simulink model "three_level_sv"  (R2025a)
settings: Solver=ode1be  StartTime=0.0  StopTime=simlength  FixedStep=ts_sim  MaxStep=ts_sim
undefined symbols (not defined in the file): fPWM_INV, number_of_cells, Q, q1Kalman, q2Kalman, q3Kalman, rKalman, tc, ts_afe, ts_zvs, tsample, Vbattery_nom
libraries: fl_lib x118, nesl_utility x60, ee_lib x3, spsPWMGenerator3LevelLib x3, lithium_ion_cell_lib x2, simulink x2
(part 1 of 4)
settings Model: SimulationMode=accelerator  Creator=LTNBDA  LastModifiedBy=dbagn
settings SolverCC: ZeroCrossControl=EnableAll  ZeroCrossAlgorithm=Adaptive  AlgebraicLoopSolver=TrustRegion  SolverResetMethod=Robust  AutoInsertRateTranBlk=on
settings DataIOCC: LimitDataPoints=on  MaxDataPoints=1  SaveFormat=Array  SignalLoggingSaveFormat=ModelDataLogs  SaveOutput=off  SignalLogging=off  DSMLogging=off  SaveTime=off  ReturnWorkspaceOutputs=off
settings OptimizationCC: ExpressionDepthLimit=2147483647.0  InitFltsAndDblsToZero=on  EfficientMapNaN2IntZero=off  LifeSpan=inf
settings DebuggingCC: SaveWithParameterizedLinksMsg=none  UnderspecifiedInitializationDetection=Classic  MergeDetectMultiDrivingBlocksExec=none  SignalResolutionControl=TryResolveAllWithWarning  SolverPrmCheckMsg=warning  MultiTaskDSMMsg=warning  MultiTaskCondExecSysMsg=none  MultiTaskRateTransMsg=warning  FcnCallInpInsideContextMsg=warning  StateNameClashWarn=warning  SFUnexpectedBacktrackingDiag=warning  SFNoUnconditionalDefaultTransitionDiag=warning  ArithmeticOperatorsInVariantConditions=warning
settings HardwareCC: ProdBitPerLong=64.0  ProdLargestAtomicFloat=None  ProdIntDivRoundTo=Undefined  ProdEndianess=Unspecified  ProdHWDeviceType=Generic->64-bit Embedded Processor (LP64)  TargetBitPerPointer=64.0  TargetBitPerSizeT=64.0  TargetBitPerPtrDiffT=64.0  TargetLongLongMode=on  TargetIntDivRoundTo=Zero  TargetEndianess=LittleEndian  TargetWordSize=64.0  TargetHWDeviceType=MATLAB Host  ProdEqTarget=off
settings ModelReferenceCC: EnableRefExpFcnMdlSchedulingChecks=on  PropagateSignalLabelsOutOfModel=off
settings SFSimCC: SimUseLocalCustomCode=off  CustomCodeUndefinedFunction=UseInterfaceOnly
settings RTWCC: RTWUseLocalCustomCode=off  GPUComputeCapability=3.5
settings CodeAppCC: MaxIdLength=128.0  StateflowObjectComments=on
settings GRTTargetCC: TargetLangStandard=C89/C90 (ANSI)  CombineOutputUpdateFcns=off  GRTInterface=on
settings ConfigComp: CovMetricSettings=dw  CovSaveCumulativeToWorkspaceVar=on  CovSaveSingleToWorkspaceVar=on  CovExternalEMLEnable=off
settings SimscapeCC: SimscapeNormalizeSystem=off

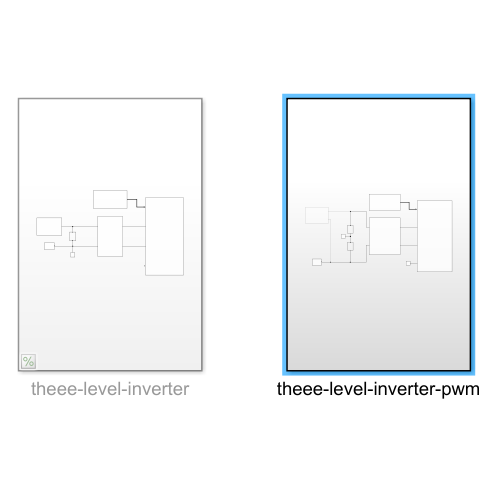
[thumbnail: Simulink's stored preview of the top-level diagram]
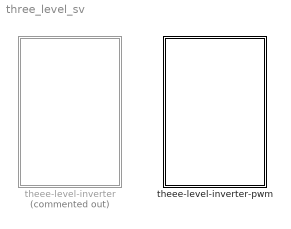
== system three_level_sv ==
  theee-level-inverter : Subsystem  Commented=on
  theee-level-inverter-pwm : Subsystem

== system three_level_sv/theee-level-inverter ==
  Electrical Reference2 : fl_lib/Electrical/Electrical Elements/Electrical Reference
  Solver Configuration : nesl_utility/Solver Configuration  PhysicalDomain=network_engine_domain  SubClassName=solver  LeftPortType=input  RightPortType=generic  Tones=[]  Harmonics=[]  SimulateNoise=off  Profile=off  UseLocalSampling=off  EnableSwitchedLinearOptims=on  FrequencyDomain=off  UseCCode=off  RelTol=0.001  AbsTol=0.001  MinStep=1e-09  ToWorkspace=off  RevertToSquareIcSolve=off  NumHomotopyIterations=100  PhasorMode=off  PhasorModeNumHarmonics=1  ConsistencySolver=NEWTON_FTOL  IndexReductionMethod=DerivativeReplacement  DoDC=on  ResidualTolerance=1e-09  ConsistencyTolSource=GLOBAL  ConsistencyAbsTol=0.001  ConsistencyRelTol=0.001  ConsistencyTolFactor=0.001  UseLocalSolver=on  LocalSolverChoice=NE_BACKWARD_EULER_ADVANCER  ResolveIndetEquations=on  FunctionEvalNumThread=1  LocalSolverSampleTime=ts_sim  DoFixedCost=on  MaxNonlinIter=3  MaxModeIter=2  ComputeImpulses=off  ImpulseIterations=2  LinearAlgebra=auto  LinearAlgebraNumThread=0  EquationFormulation=NE_TIME_EF  DelaysMemoryBudget=1024  AutomaticFiltering=on  FilteringTimeConstant=0.001  PartitionStorageMethod=AS_NEEDED  PartitionMemoryBudget=1024  PartitionMethod=ROBUST  MultibodyUseLocalSolver=off  MultibodyLocalSolverChoice=ODE1  MultibodyLocalSolverSampleTime=0.001
  Voltage Source : ee_lib/Sources/Voltage Source  dc_voltage=Vbattery_nom V  ac_voltage=0 V  ac_shift=0 rad  ac_frequency=60 Hz  noise_mode=ee.enum.sources.noise.Disabled  PSD=0 V^2/Hz  sample_time=1e-3 s  repeatability=ee.enum.sources.repeatability.NotRepeatable  user_seed=0  auto_seed=3499211588  i_specify=off  i_priority=None  i=0 A  i_nominal_specify=off  i_nominal_value=1  i_nominal_unit=A  v_specify=off  v_priority=None  v=0 V  v_nominal_specify=off  v_nominal_value=1  v_nominal_unit=V
  battery_system : Subsystem
  pwm_commands : Subsystem
  single_phase_ui_measure1 : Subsystem
  three-level-inverter : Subsystem
  wires:
  pwm_commands/1(gate_commands) -> three-level-inverter/1(gate_commands)
  connections:
  three-level-inverter/LConn2 -- single_phase_ui_measure1/RConn2
  battery_system/RConn1 -- Voltage Source/LConn1 -- single_phase_ui_measure1/LConn1
  single_phase_ui_measure1/RConn1 -- three-level-inverter/LConn1
  single_phase_ui_measure1/LConn2 -- Electrical Reference2/LConn1 -- Voltage Source/RConn1 -- Solver Configuration/RConn1

== system three_level_sv/theee-level-inverter-pwm ==
  Electrical Reference1 : fl_lib/Electrical/Electrical Elements/Electrical Reference
  Electrical Reference2 : fl_lib/Electrical/Electrical Elements/Electrical Reference
  Solver Configuration : nesl_utility/Solver Configuration  PhysicalDomain=network_engine_domain  SubClassName=solver  LeftPortType=input  RightPortType=generic  Tones=[]  Harmonics=[]  SimulateNoise=off  Profile=off  UseLocalSampling=off  EnableSwitchedLinearOptims=on  FrequencyDomain=off  UseCCode=off  RelTol=0.001  AbsTol=0.001  MinStep=1e-09  ToWorkspace=off  RevertToSquareIcSolve=off  NumHomotopyIterations=100  PhasorMode=off  PhasorModeNumHarmonics=1  ConsistencySolver=NEWTON_FTOL  IndexReductionMethod=DerivativeReplacement  DoDC=on  ResidualTolerance=1e-09  ConsistencyTolSource=GLOBAL  ConsistencyAbsTol=0.001  ConsistencyRelTol=0.001  ConsistencyTolFactor=0.001  UseLocalSolver=on  LocalSolverChoice=NE_BACKWARD_EULER_ADVANCER  ResolveIndetEquations=on  FunctionEvalNumThread=1  LocalSolverSampleTime=ts_sim  DoFixedCost=on  MaxNonlinIter=3  MaxModeIter=2  ComputeImpulses=off  ImpulseIterations=2  LinearAlgebra=auto  LinearAlgebraNumThread=0  EquationFormulation=NE_TIME_EF  DelaysMemoryBudget=1024  AutomaticFiltering=on  FilteringTimeConstant=0.001  PartitionStorageMethod=AS_NEEDED  PartitionMemoryBudget=1024  PartitionMethod=ROBUST  MultibodyUseLocalSolver=off  MultibodyLocalSolverChoice=ODE1  MultibodyLocalSolverSampleTime=0.001
  Voltage Source : ee_lib/Sources/Voltage Source  dc_voltage=Vbattery_nom/2 V  ac_voltage=0 V  ac_shift=0 rad  ac_frequency=60 Hz  noise_mode=ee.enum.sources.noise.Disabled  PSD=0 V^2/Hz  sample_time=1e-3 s  repeatability=ee.enum.sources.repeatability.NotRepeatable  user_seed=0  auto_seed=3499211588  i_specify=off  i_priority=None  i=0 A  i_nominal_specify=off  i_nominal_value=1  i_nominal_unit=A  v_specify=off  v_priority=None  v=0 V  v_nominal_specify=off  v_nominal_value=1  v_nominal_unit=V
  Voltage Source1 : ee_lib/Sources/Voltage Source  dc_voltage=Vbattery_nom/2 V  ac_voltage=0 V  ac_shift=0 rad  ac_frequency=60 Hz  noise_mode=ee.enum.sources.noise.Disabled  PSD=0 V^2/Hz  sample_time=1e-3 s  repeatability=ee.enum.sources.repeatability.NotRepeatable  user_seed=0  auto_seed=545404223  i_specify=off  i_priority=None  i=0 A  i_nominal_specify=off  i_nominal_value=1  i_nominal_unit=A  v_specify=off  v_priority=None  v=0 V  v_nominal_specify=off  v_nominal_value=1  v_nominal_unit=V
  battery_system : Subsystem  Commented=on
  pwm_commands : Subsystem
  single_phase_ui_measure1 : Subsystem
  three-level-inverter : Subsystem
  wires:
  pwm_commands/1(gate_commands) -> three-level-inverter/1(gate_commands)
  connections:
  Voltage Source1/RConn1 -- single_phase_ui_measure1/LConn2 -- battery_system/RConn2 -- Solver Configuration/RConn1
  single_phase_ui_measure1/RConn1 -- three-level-inverter/LConn1
  single_phase_ui_measure1/LConn1 -- Voltage Source/LConn1 -- battery_system/RConn1
  three-level-inverter/LConn2 -- single_phase_ui_measure1/RConn2
  Electrical Reference2/LConn1 -- three-level-inverter/LConn3
  Voltage Source1/LConn1 -- Electrical Reference1/LConn1 -- Voltage Source/RConn1

== system three_level_sv/theee-level-inverter/battery_system ==
  Electrical Reference1 : fl_lib/Electrical/Electrical Elements/Electrical Reference
  LithiumIonBattery : Subsystem
  Uout+ : PMIOPort  Side=Right
  connections:
  LithiumIonBattery/RConn2 -- Electrical Reference1/LConn1
  LithiumIonBattery/RConn1 -- Uout+/RConn1

== system three_level_sv/theee-level-inverter/pwm_commands ==
  Demux : Demux  Outputs=3
  Gain12 : Gain  Gain=eye(12)  Multiplication=Matrix(u*K)
  Manual Switch : ManualSwitch
  XY Graph : Record  NumPorts=2.0  FileSettingsInternal="{\"entries\":[{\"content\":{\"excelSettings\":{\"content\":{},\"type\":\"Streamout.ExcelSettings\"},\"parquetSettings\":{\"content\":{},\"type\":\"Streamout.ParquetSettings\"}},\"type\":\"Streamout.FileSettingStorage\",\"uuid\":\"\"}],\"packageUris\":[\"http:\\/\\/schema.mathworks.com\\/mf0\\/streamout_blocks\\/R2020a\"],\"version\":\"1.0\"}"  FrameSettings=[0, 0]  Layout=[1 1]  SignalsInternal="{\"entries\":[{\"content\":{},\"type\":\"RecordBlkView.InputSignals\",\"uuid\":\"\"}],\"packageUris\":[\"http:\\/\\/schema.mathworks.com\\/mf0\\/streamout_blocks\\/R2020a\"],\"version\":\"1.0\"}"  VisualizationBindings="{\"xyplotplugin\":{\"info\":[{\"series\":[],\"subplotID\":1}]}}"  CompatibilityTag=XY
  abc2alphabeta : MATLAB Function  TreatAsAtomicUnit=on  SystemSampleTime=ts_afe
  counter_12 : MATLAB Function  TreatAsAtomicUnit=on  SystemSampleTime=500e-6  mask{Nmax=12}
  counter_6 : MATLAB Function  TreatAsAtomicUnit=on  SystemSampleTime=1e-3  mask{Nmax=6}
  counters : Scope  NumInputPorts=2
      settings: ActiveDisplayYMinimum=-0.375  ActiveDisplayYMaximum=13.375
  index2sv_12 : MATLAB Function  TreatAsAtomicUnit=on  SystemSampleTime=ts_afe
  index2sv_6 : MATLAB Function  TreatAsAtomicUnit=on  SystemSampleTime=ts_afe
  sv2gata_cmds : MATLAB Function  TreatAsAtomicUnit=on  SystemSampleTime=ts_afe
  gate_commands : Outport
  wires:
  sv2gata_cmds/1(y) -> Gain12/1
  Gain12/1 -> gate_commands/1
  counter_6/1(y) -> index2sv_6/1(i), counters/1
  Demux/1 -> abc2alphabeta/1(u)
  Demux/2 -> abc2alphabeta/2(v)
  Demux/3 -> abc2alphabeta/3(w)
  abc2alphabeta/1(alpha) -> XY Graph/1
  abc2alphabeta/2(beta) -> XY Graph/2
  counter_12/1(y) -> counters/2, index2sv_12/1(i)
  Manual Switch/1 -> Demux/1, sv2gata_cmds/1(u)
  index2sv_6/1(y) -> Manual Switch/2
  index2sv_12/1(y) -> Manual Switch/1

== system three_level_sv/theee-level-inverter/single_phase_ui_measure1 ==
  Bus Creator : BusCreator  Inputs=2
  Current Sensor : fl_lib/Electrical/Electrical Sensors/Current Sensor
  Selector : Selector  InputPortWidth=2  IndexOptions=Index vector (dialog)  Indices=2  OutputSizes=1
  Selector1 : Selector  InputPortWidth=2  IndexOptions=Index vector (dialog)  Indices=1  OutputSizes=1
  Voltage Sensor : fl_lib/Electrical/Electrical Sensors/Voltage Sensor
  input : Scope  NumInputPorts=2
      settings: SampleTime=tc  ActiveDisplayYMinimum=-46.7569  ActiveDisplayYMaximum=366.3097  DataLoggingVariableName=ScopeData2
  iph : nesl_utility/PS-Simulink Converter  PhysicalDomain=network_engine_domain  SubClassName=ps_output  LeftPortType=input  RightPortType=output  PseudoPeriodic=off  Frequencies=[]  VectorFormat=1-D array  Unit=A  AffineConversion=off
  uph : nesl_utility/PS-Simulink Converter  PhysicalDomain=network_engine_domain  SubClassName=ps_output  LeftPortType=input  RightPortType=output  PseudoPeriodic=off  Frequencies=[]  VectorFormat=1-D array  Unit=V  AffineConversion=off
  Udc(+) : PMIOPort  Side=Left
  udc(+) : PMIOPort  Port=2  Side=Right
  Udc(-) : PMIOPort  Port=3  Side=Left
  udc(-) : PMIOPort  Port=4  Side=Right
  tag scope: current_battery=global, voltage_battery=global
  wires:
  Bus Creator/1 -> Selector/1, Selector1/1  "ui_data"
  iph/1 -> Bus Creator/1  "iph"
  uph/1 -> Bus Creator/2  "uph"
  Selector1/1 -> [current_battery], input/1  "current_battery"
  Selector/1 -> input/2, [voltage_battery]  "voltage_battery"
  connections:
  iph/LConn1 -- Current Sensor/RConn1
  Voltage Sensor/LConn1 -- Current Sensor/LConn1 -- Udc(+)/RConn1
  Current Sensor/RConn2 -- udc(+)/RConn1
  Voltage Sensor/RConn1 -- uph/LConn1
  Voltage Sensor/RConn2 -- Udc(-)/RConn1 -- udc(-)/RConn1

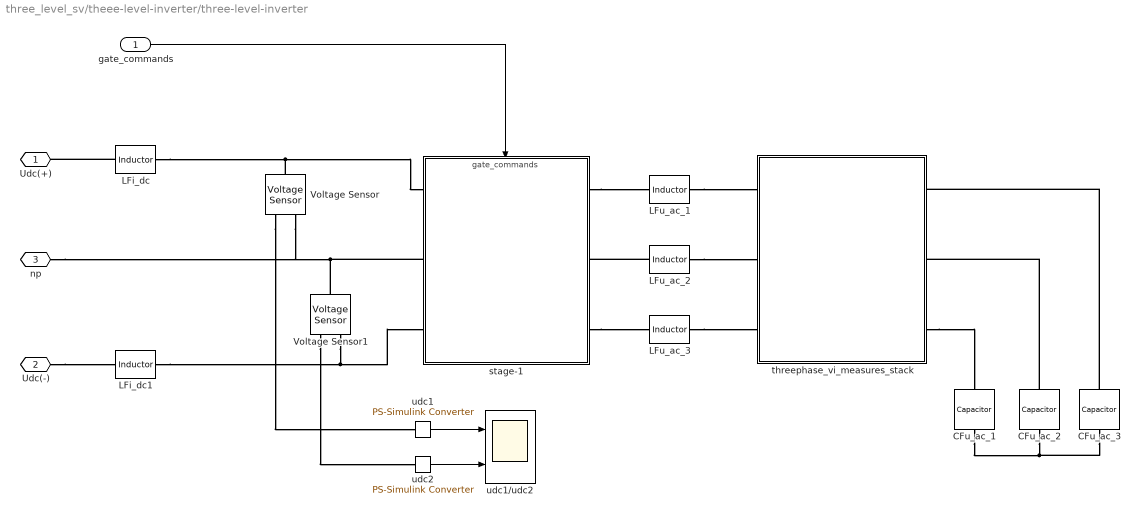
== system three_level_sv/theee-level-inverter/three-level-inverter ==
  gate_commands : Inport
  CFu_ac_1 : fl_lib/Electrical/Electrical Elements/Capacitor  c=400e-6 F  r=100e-3 Ohm  g=0 1/Ohm  i_specify=off  i_priority=None  i=0 A  i_nominal_specify=off  i_nominal_value=1  i_nominal_unit=A  v_specify=off  v_priority=None  v=0 V  v_nominal_specify=off  v_nominal_value=1  v_nominal_unit=V  vc_specify=off  vc_priority=High  vc=0 V  vc_nominal_specify=off  vc_nominal_value=1  vc_nominal_unit=V
  CFu_ac_2 : fl_lib/Electrical/Electrical Elements/Capacitor  c=400e-6 F  r=100e-3 Ohm  g=0 1/Ohm  i_specify=off  i_priority=None  i=0 A  i_nominal_specify=off  i_nominal_value=1  i_nominal_unit=A  v_specify=off  v_priority=None  v=0 V  v_nominal_specify=off  v_nominal_value=1  v_nominal_unit=V  vc_specify=off  vc_priority=High  vc=0 V  vc_nominal_specify=off  vc_nominal_value=1  vc_nominal_unit=V
  CFu_ac_3 : fl_lib/Electrical/Electrical Elements/Capacitor  c=400e-6 F  r=100e-3 Ohm  g=0 1/Ohm  i_specify=off  i_priority=None  i=0 A  i_nominal_specify=off  i_nominal_value=1  i_nominal_unit=A  v_specify=off  v_priority=None  v=0 V  v_nominal_specify=off  v_nominal_value=1  v_nominal_unit=V  vc_specify=off  vc_priority=High  vc=0 V  vc_nominal_specify=off  vc_nominal_value=1  vc_nominal_unit=V
  LFi_dc : fl_lib/Electrical/Electrical Elements/Inductor  l=150e-6 H  r=0 Ohm  g=1e-9 1/Ohm  i_specify=off  i_priority=None  i=0 A  i_nominal_specify=off  i_nominal_value=1  i_nominal_unit=A  v_specify=off  v_priority=None  v=0 V  v_nominal_specify=off  v_nominal_value=1  v_nominal_unit=V  i_L_specify=off  i_L_priority=High  i_L=0 A  i_L_nominal_specify=off  i_L_nominal_value=1  i_L_nominal_unit=A
  LFi_dc1 : fl_lib/Electrical/Electrical Elements/Inductor  l=150e-6 H  r=0 Ohm  g=1e-9 1/Ohm  i_specify=off  i_priority=None  i=0 A  i_nominal_specify=off  i_nominal_value=1  i_nominal_unit=A  v_specify=off  v_priority=None  v=0 V  v_nominal_specify=off  v_nominal_value=1  v_nominal_unit=V  i_L_specify=off  i_L_priority=High  i_L=0 A  i_L_nominal_specify=off  i_L_nominal_value=1  i_L_nominal_unit=A
  LFu_ac_1 : fl_lib/Electrical/Electrical Elements/Inductor  l=250e-6 H  r=3e-3 Ohm  g=1e-9 1/Ohm  i_specify=off  i_priority=None  i=0 A  i_nominal_specify=off  i_nominal_value=1  i_nominal_unit=A  v_specify=off  v_priority=None  v=0 V  v_nominal_specify=off  v_nominal_value=1  v_nominal_unit=V  i_L_specify=off  i_L_priority=High  i_L=0 A  i_L_nominal_specify=off  i_L_nominal_value=1  i_L_nominal_unit=A
  LFu_ac_2 : fl_lib/Electrical/Electrical Elements/Inductor  l=250e-6 H  r=3e-3 Ohm  g=1e-9 1/Ohm  i_specify=off  i_priority=None  i=0 A  i_nominal_specify=off  i_nominal_value=1  i_nominal_unit=A  v_specify=off  v_priority=None  v=0 V  v_nominal_specify=off  v_nominal_value=1  v_nominal_unit=V  i_L_specify=off  i_L_priority=High  i_L=0 A  i_L_nominal_specify=off  i_L_nominal_value=1  i_L_nominal_unit=A
  LFu_ac_3 : fl_lib/Electrical/Electrical Elements/Inductor  l=250e-6 H  r=3e-3 Ohm  g=1e-9 1/Ohm  i_specify=off  i_priority=None  i=0 A  i_nominal_specify=off  i_nominal_value=1  i_nominal_unit=A  v_specify=off  v_priority=None  v=0 V  v_nominal_specify=off  v_nominal_value=1  v_nominal_unit=V  i_L_specify=off  i_L_priority=High  i_L=0 A  i_L_nominal_specify=off  i_L_nominal_value=1  i_L_nominal_unit=A
  Voltage Sensor : fl_lib/Electrical/Electrical Sensors/Voltage Sensor
  Voltage Sensor1 : fl_lib/Electrical/Electrical Sensors/Voltage Sensor
  stage-1 : Subsystem
      settings: PortSchema="{\"entries\":[{\"content\":{\"sides\":[{\"content\":{\"connectorIds\":[\"LConn1\",\"LConn2\",\"LConn3\"]},\"type\":\"ConnectorPlacement.EquallySpacedRectSide\",\"uuid\":\"c872503a-61af-4937-bdf2-4de4f8645573\"},{\"content\":{\"connectorIds\":[\"RConn1\",\"RConn2\",\"RConn3\"],\"side\":\"RIGHT\"},\"type\":\"ConnectorPlacement.EquallySpacedRectSide\",\"uuid\":\"3b83f060-86a2-4569-84b5-d9f7c0485347\"},{\"content\":{\"connectorIds\":[\"In1\"],\"side\":\"TOP\"},\"type\":\"ConnectorPlacement.EquallySpacedRectSide\",\"uuid\":\"bf191d46-ce71-4d15-9dd0-24cc57253577\"}]},\"type\":\"ConnectorPlacement.EquallySpacedConnector\",\"uuid\":\"1b28ceee-25d0-45ae-a3c4-c2563f0d63ba\"}],\"packageUris\":[\"http://schema.mathworks.com/mf0/Connector/R2020b\"],\"version\":\"1.0\"}"
  threephase_vi_measures_stack : Subsystem
  udc1 : nesl_utility/PS-Simulink Converter  PhysicalDomain=network_engine_domain  SubClassName=ps_output  LeftPortType=input  RightPortType=output  PseudoPeriodic=off  Frequencies=[]  VectorFormat=1-D array  Unit=V  AffineConversion=off
  udc1/udc2 : Scope  NumInputPorts=2
      settings: SampleTime=tc  ActiveDisplayYMinimum=50.31273  ActiveDisplayYMaximum=57.5418  DataLoggingVariableName=ScopeData5
  udc2 : nesl_utility/PS-Simulink Converter  PhysicalDomain=network_engine_domain  SubClassName=ps_output  LeftPortType=input  RightPortType=output  PseudoPeriodic=off  Frequencies=[]  VectorFormat=1-D array  Unit=V  AffineConversion=off
  Udc(+) : PMIOPort  Side=Left
  Udc(-) : PMIOPort  Port=2  Side=Left
  np : PMIOPort  Port=3  Side=Left
  wires:
  gate_commands/1 -> stage-1/1(gate_commands)
  udc1/1 -> udc1/udc2/1
  udc2/1 -> udc1/udc2/2
  connections:
  LFi_dc/LConn1 -- Udc(+)/RConn1
  LFi_dc/RConn1 -- stage-1/RConn1 -- Voltage Sensor/LConn1
  CFu_ac_1/RConn1 -- CFu_ac_3/RConn1 -- CFu_ac_2/RConn1
  LFu_ac_2/LConn1 -- stage-1/LConn2
  stage-1/LConn1 -- LFu_ac_1/LConn1
  stage-1/LConn3 -- LFu_ac_3/LConn1
  LFu_ac_1/RConn1 -- threephase_vi_measures_stack/LConn1
  LFu_ac_2/RConn1 -- threephase_vi_measures_stack/LConn2
  LFu_ac_3/RConn1 -- threephase_vi_measures_stack/LConn3
  threephase_vi_measures_stack/RConn3 -- CFu_ac_1/LConn1
  CFu_ac_2/LConn1 -- threephase_vi_measures_stack/RConn2
  CFu_ac_3/LConn1 -- threephase_vi_measures_stack/RConn1
  Voltage Sensor1/RConn1 -- udc2/LConn1
  Voltage Sensor/RConn1 -- udc1/LConn1
  LFi_dc1/RConn1 -- Voltage Sensor1/RConn2 -- stage-1/RConn3
  stage-1/RConn2 -- np/RConn1 -- Voltage Sensor/RConn2 -- Voltage Sensor1/LConn1
  Udc(-)/RConn1 -- LFi_dc1/LConn1

== system three_level_sv/theee-level-inverter-pwm/battery_system ==
  LithiumIonBattery : Subsystem
  Uout+ : PMIOPort  Side=Right
  Uout- : PMIOPort  Port=2  Side=Right
  connections:
  LithiumIonBattery/RConn1 -- Uout+/RConn1
  LithiumIonBattery/RConn2 -- Uout-/RConn1

== system three_level_sv/theee-level-inverter-pwm/pwm_commands ==
  Constant : Constant  Value=0
  Mux1 : Mux  Inputs=3
  Mux2 : Mux  Inputs=3
  PWM Generator (3-Level)3 : spsPWMGenerator3LevelLib/PWM Generator (3-Level)  ModulatorType=Single-phase half-bridge (4 pulses)  ModulatorMode=Unsynchronized  nF=27  Fc=fPWM_INV  ModulatingSignals=off  m=0.8  Freq=50  Phase=0  Ts=0
      settings: LibrarySourceBlock=|
      | sps_lib/Power Electronics/Power Electronics Control/PWM Generator
      | (3-Level)
  PWM Generator (3-Level)5 : spsPWMGenerator3LevelLib/PWM Generator (3-Level)  ModulatorType=Single-phase half-bridge (4 pulses)  ModulatorMode=Unsynchronized  nF=27  Fc=fPWM_INV  ModulatingSignals=off  m=0.8  Freq=50  Phase=0  Ts=0
      settings: LibrarySourceBlock=|
      | sps_lib/Power Electronics/Power Electronics Control/PWM Generator
      | (3-Level)
  PWM Generator (3-Level)6 : spsPWMGenerator3LevelLib/PWM Generator (3-Level)  ModulatorType=Single-phase half-bridge (4 pulses)  ModulatorMode=Unsynchronized  nF=27  Fc=fPWM_INV  ModulatingSignals=off  m=0.8  Freq=50  Phase=0  Ts=0
      settings: LibrarySourceBlock=|
      | sps_lib/Power Electronics/Power Electronics Control/PWM Generator
      | (3-Level)
  PWM generator u : Subsystem  Commented=on  mask{f=fPWM_INV, m_up=1, m_low=-1, dead_time=0, pos_cmd_gate=1, neg_cmd_gate=0, polarity=1}
      mask prompts: f "Frequency (Hz)"; m_up "Max Input Modulation Value"; m_low "Min Input Modulation Value"; dead_time "Dead Time (s)"; pos_cmd_gate "Positive Gate Voltage (V)"; neg_cmd_gate "Negative Gate Voltage (V)"; polarity "Polarity (pu)"
  PWM generator u1 : Subsystem  Commented=on  mask{f=fPWM_INV, m_up=1, m_low=-1, dead_time=0, pos_cmd_gate=1, neg_cmd_gate=0, polarity=1}
      mask prompts: f "Frequency (Hz)"; m_up "Max Input Modulation Value"; m_low "Min Input Modulation Value"; dead_time "Dead Time (s)"; pos_cmd_gate "Positive Gate Voltage (V)"; neg_cmd_gate "Negative Gate Voltage (V)"; polarity "Polarity (pu)"
  PWM generator u2 : Subsystem  Commented=on  mask{f=fPWM_INV, m_up=1, m_low=-1, dead_time=0, pos_cmd_gate=1, neg_cmd_gate=0, polarity=1}
      mask prompts: f "Frequency (Hz)"; m_up "Max Input Modulation Value"; m_low "Min Input Modulation Value"; dead_time "Dead Time (s)"; pos_cmd_gate "Positive Gate Voltage (V)"; neg_cmd_gate "Negative Gate Voltage (V)"; polarity "Polarity (pu)"
  Sine Wave : Sin  Amplitude=0.8  Frequency=2*pi*50  SampleTime=0
  Sine Wave1 : Sin  Amplitude=0.8  Frequency=2*pi*50  Phase=-2*pi/3  SampleTime=0
  Sine Wave2 : Sin  Amplitude=0.8  Frequency=2*pi*50  Phase=2*pi/3  SampleTime=0
  gate_commands : Outport
  wires:
  PWM Generator (3-Level)3/1 -> Mux1/2  "PWM generator v"
  PWM Generator (3-Level)6/1 -> Mux1/1  "PWM generator u"
  PWM Generator (3-Level)5/1 -> Mux1/3  "PWM generator w"
  Sine Wave/1 -> PWM generator u/1(m_index), PWM Generator (3-Level)6/1
  Sine Wave1/1 -> PWM generator u1/1(m_index), PWM Generator (3-Level)3/1
  Sine Wave2/1 -> PWM generator u2/1(m_index), PWM Generator (3-Level)5/1
  PWM generator u1/1(m) -> Mux2/2  "PWM generator v"
  PWM generator u/1(m) -> Mux2/1  "PWM generator u"
  PWM generator u2/1(m) -> Mux2/3  "PWM generator w"
  Constant/1 -> PWM generator u/2(phase), PWM generator u1/2(phase), PWM generator u2/2(phase)
  Mux1/1 -> gate_commands/1

== system three_level_sv/theee-level-inverter-pwm/single_phase_ui_measure1 ==
  Bus Creator : BusCreator  Inputs=2
  Current Sensor : fl_lib/Electrical/Electrical Sensors/Current Sensor
  Selector : Selector  InputPortWidth=2  IndexOptions=Index vector (dialog)  Indices=2  OutputSizes=1
  Selector1 : Selector  InputPortWidth=2  IndexOptions=Index vector (dialog)  Indices=1  OutputSizes=1
  Voltage Sensor : fl_lib/Electrical/Electrical Sensors/Voltage Sensor
  input : Scope  NumInputPorts=2
      settings: SampleTime=tc  ActiveDisplayYMinimum=-33.484772411535481  ActiveDisplayYMaximum=36.300700209973051  DataLoggingVariableName=ScopeData2
  iph : nesl_utility/PS-Simulink Converter  PhysicalDomain=network_engine_domain  SubClassName=ps_output  LeftPortType=input  RightPortType=output  PseudoPeriodic=off  Frequencies=[]  VectorFormat=1-D array  Unit=A  AffineConversion=off
  uph : nesl_utility/PS-Simulink Converter  PhysicalDomain=network_engine_domain  SubClassName=ps_output  LeftPortType=input  RightPortType=output  PseudoPeriodic=off  Frequencies=[]  VectorFormat=1-D array  Unit=V  AffineConversion=off
  Udc(+) : PMIOPort  Side=Left
  udc(+) : PMIOPort  Port=2  Side=Right
  Udc(-) : PMIOPort  Port=3  Side=Left
  udc(-) : PMIOPort  Port=4  Side=Right
  tag scope: current_battery=global, voltage_battery=global
  wires:
  Selector/1 -> [voltage_battery], input/2  "voltage_battery"
  Selector1/1 -> input/1, [current_battery]  "current_battery"
  uph/1 -> Bus Creator/2  "uph"
  iph/1 -> Bus Creator/1  "iph"
  Bus Creator/1 -> Selector1/1, Selector/1  "ui_data"
  connections:
  udc(-)/RConn1 -- Udc(-)/RConn1 -- Voltage Sensor/RConn2
  Voltage Sensor/RConn1 -- uph/LConn1
  Current Sensor/RConn2 -- udc(+)/RConn1
  Udc(+)/RConn1 -- Current Sensor/LConn1 -- Voltage Sensor/LConn1
  iph/LConn1 -- Current Sensor/RConn1

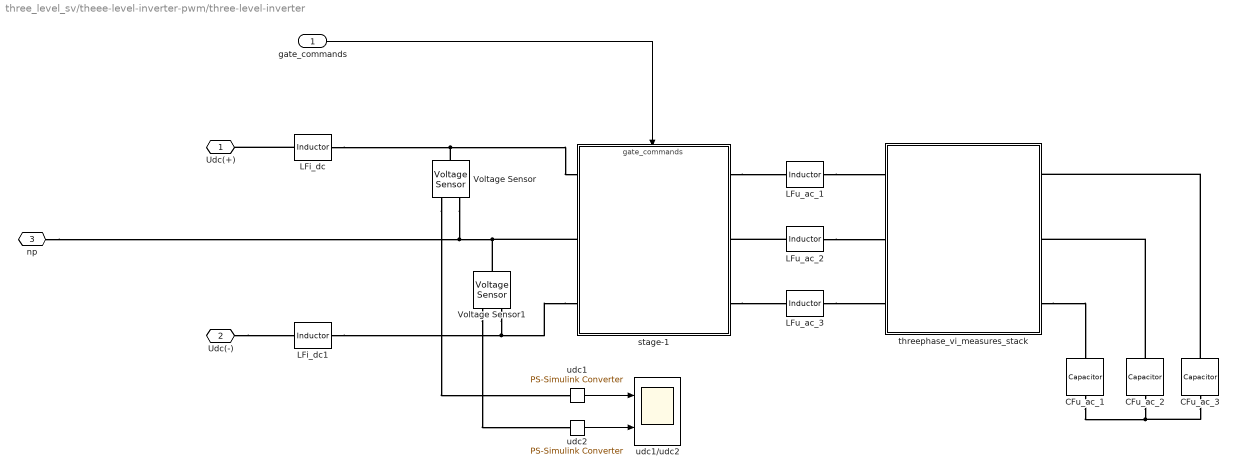
== system three_level_sv/theee-level-inverter-pwm/three-level-inverter ==
  gate_commands : Inport
  CFu_ac_1 : fl_lib/Electrical/Electrical Elements/Capacitor  c=400e-6 F  r=100e-3 Ohm  g=0 1/Ohm  i_specify=off  i_priority=None  i=0 A  i_nominal_specify=off  i_nominal_value=1  i_nominal_unit=A  v_specify=off  v_priority=None  v=0 V  v_nominal_specify=off  v_nominal_value=1  v_nominal_unit=V  vc_specify=off  vc_priority=High  vc=0 V  vc_nominal_specify=off  vc_nominal_value=1  vc_nominal_unit=V
  CFu_ac_2 : fl_lib/Electrical/Electrical Elements/Capacitor  c=400e-6 F  r=100e-3 Ohm  g=0 1/Ohm  i_specify=off  i_priority=None  i=0 A  i_nominal_specify=off  i_nominal_value=1  i_nominal_unit=A  v_specify=off  v_priority=None  v=0 V  v_nominal_specify=off  v_nominal_value=1  v_nominal_unit=V  vc_specify=off  vc_priority=High  vc=0 V  vc_nominal_specify=off  vc_nominal_value=1  vc_nominal_unit=V
  CFu_ac_3 : fl_lib/Electrical/Electrical Elements/Capacitor  c=400e-6 F  r=100e-3 Ohm  g=0 1/Ohm  i_specify=off  i_priority=None  i=0 A  i_nominal_specify=off  i_nominal_value=1  i_nominal_unit=A  v_specify=off  v_priority=None  v=0 V  v_nominal_specify=off  v_nominal_value=1  v_nominal_unit=V  vc_specify=off  vc_priority=High  vc=0 V  vc_nominal_specify=off  vc_nominal_value=1  vc_nominal_unit=V
  LFi_dc : fl_lib/Electrical/Electrical Elements/Inductor  l=150e-6 H  r=0 Ohm  g=1e-9 1/Ohm  i_specify=off  i_priority=None  i=0 A  i_nominal_specify=off  i_nominal_value=1  i_nominal_unit=A  v_specify=off  v_priority=None  v=0 V  v_nominal_specify=off  v_nominal_value=1  v_nominal_unit=V  i_L_specify=off  i_L_priority=High  i_L=0 A  i_L_nominal_specify=off  i_L_nominal_value=1  i_L_nominal_unit=A
  LFi_dc1 : fl_lib/Electrical/Electrical Elements/Inductor  l=150e-6 H  r=0 Ohm  g=1e-9 1/Ohm  i_specify=off  i_priority=None  i=0 A  i_nominal_specify=off  i_nominal_value=1  i_nominal_unit=A  v_specify=off  v_priority=None  v=0 V  v_nominal_specify=off  v_nominal_value=1  v_nominal_unit=V  i_L_specify=off  i_L_priority=High  i_L=0 A  i_L_nominal_specify=off  i_L_nominal_value=1  i_L_nominal_unit=A
  LFu_ac_1 : fl_lib/Electrical/Electrical Elements/Inductor  l=250e-6 H  r=3e-3 Ohm  g=1e-9 1/Ohm  i_specify=off  i_priority=None  i=0 A  i_nominal_specify=off  i_nominal_value=1  i_nominal_unit=A  v_specify=off  v_priority=None  v=0 V  v_nominal_specify=off  v_nominal_value=1  v_nominal_unit=V  i_L_specify=off  i_L_priority=High  i_L=0 A  i_L_nominal_specify=off  i_L_nominal_value=1  i_L_nominal_unit=A
  LFu_ac_2 : fl_lib/Electrical/Electrical Elements/Inductor  l=250e-6 H  r=3e-3 Ohm  g=1e-9 1/Ohm  i_specify=off  i_priority=None  i=0 A  i_nominal_specify=off  i_nominal_value=1  i_nominal_unit=A  v_specify=off  v_priority=None  v=0 V  v_nominal_specify=off  v_nominal_value=1  v_nominal_unit=V  i_L_specify=off  i_L_priority=High  i_L=0 A  i_L_nominal_specify=off  i_L_nominal_value=1  i_L_nominal_unit=A
  LFu_ac_3 : fl_lib/Electrical/Electrical Elements/Inductor  l=250e-6 H  r=3e-3 Ohm  g=1e-9 1/Ohm  i_specify=off  i_priority=None  i=0 A  i_nominal_specify=off  i_nominal_value=1  i_nominal_unit=A  v_specify=off  v_priority=None  v=0 V  v_nominal_specify=off  v_nominal_value=1  v_nominal_unit=V  i_L_specify=off  i_L_priority=High  i_L=0 A  i_L_nominal_specify=off  i_L_nominal_value=1  i_L_nominal_unit=A
  Voltage Sensor : fl_lib/Electrical/Electrical Sensors/Voltage Sensor
  Voltage Sensor1 : fl_lib/Electrical/Electrical Sensors/Voltage Sensor
  stage-1 : Subsystem
      settings: PortSchema="{\"entries\":[{\"content\":{\"sides\":[{\"content\":{\"connectorIds\":[\"LConn1\",\"LConn2\",\"LConn3\"]},\"type\":\"ConnectorPlacement.EquallySpacedRectSide\",\"uuid\":\"c872503a-61af-4937-bdf2-4de4f8645573\"},{\"content\":{\"connectorIds\":[\"RConn1\",\"RConn2\",\"RConn3\"],\"side\":\"RIGHT\"},\"type\":\"ConnectorPlacement.EquallySpacedRectSide\",\"uuid\":\"3b83f060-86a2-4569-84b5-d9f7c0485347\"},{\"content\":{\"connectorIds\":[\"In1\"],\"side\":\"TOP\"},\"type\":\"ConnectorPlacement.EquallySpacedRectSide\",\"uuid\":\"bf191d46-ce71-4d15-9dd0-24cc57253577\"}]},\"type\":\"ConnectorPlacement.EquallySpacedConnector\",\"uuid\":\"1b28ceee-25d0-45ae-a3c4-c2563f0d63ba\"}],\"packageUris\":[\"http://schema.mathworks.com/mf0/Connector/R2020b\"],\"version\":\"1.0\"}"
  threephase_vi_measures_stack : Subsystem
  udc1 : nesl_utility/PS-Simulink Converter  PhysicalDomain=network_engine_domain  SubClassName=ps_output  LeftPortType=input  RightPortType=output  PseudoPeriodic=off  Frequencies=[]  VectorFormat=1-D array  Unit=V  AffineConversion=off
  udc1/udc2 : Scope  NumInputPorts=2
      settings: SampleTime=tc  ActiveDisplayYMinimum=98.193775469723775  ActiveDisplayYMaximum=871.15088296038266  DataLoggingVariableName=ScopeData5
  udc2 : nesl_utility/PS-Simulink Converter  PhysicalDomain=network_engine_domain  SubClassName=ps_output  LeftPortType=input  RightPortType=output  PseudoPeriodic=off  Frequencies=[]  VectorFormat=1-D array  Unit=V  AffineConversion=off
  Udc(+) : PMIOPort  Side=Left
  Udc(-) : PMIOPort  Port=2  Side=Left
  np : PMIOPort  Port=3  Side=Left
  wires:
  udc2/1 -> udc1/udc2/2
  udc1/1 -> udc1/udc2/1
  gate_commands/1 -> stage-1/1(gate_commands)
  connections:
  Udc(-)/RConn1 -- LFi_dc1/LConn1
  stage-1/RConn3 -- Voltage Sensor1/RConn2 -- LFi_dc1/RConn1
  Voltage Sensor/RConn1 -- udc1/LConn1
  Voltage Sensor1/RConn1 -- udc2/LConn1
  CFu_ac_3/LConn1 -- threephase_vi_measures_stack/RConn1
  CFu_ac_2/LConn1 -- threephase_vi_measures_stack/RConn2
  threephase_vi_measures_stack/RConn3 -- CFu_ac_1/LConn1
  LFu_ac_3/RConn1 -- threephase_vi_measures_stack/LConn3
  LFu_ac_2/RConn1 -- threephase_vi_measures_stack/LConn2
  LFu_ac_1/RConn1 -- threephase_vi_measures_stack/LConn1
  stage-1/LConn3 -- LFu_ac_3/LConn1
  stage-1/LConn1 -- LFu_ac_1/LConn1
  LFu_ac_2/LConn1 -- stage-1/LConn2
  Voltage Sensor1/LConn1 -- np/RConn1 -- Voltage Sensor/RConn2 -- stage-1/RConn2
  Voltage Sensor/LConn1 -- stage-1/RConn1 -- LFi_dc/RConn1
  LFi_dc/LConn1 -- Udc(+)/RConn1
  CFu_ac_2/RConn1 -- CFu_ac_1/RConn1 -- CFu_ac_3/RConn1

== system three_level_sv/theee-level-inverter/battery_system/LithiumIonBattery ==
  Current Sensor : fl_lib/Electrical/Electrical Sensors/Current Sensor
  Electrical Reference1 : fl_lib/Electrical/Electrical Elements/Electrical Reference
  PS-Simulink Converter4 : nesl_utility/PS-Simulink Converter  PhysicalDomain=network_engine_domain  SubClassName=ps_output  LeftPortType=input  RightPortType=output  PseudoPeriodic=off  Frequencies=[]  VectorFormat=1-D array  Unit=1  AffineConversion=off
  PS-Simulink Converter5 : nesl_utility/PS-Simulink Converter  PhysicalDomain=network_engine_domain  SubClassName=ps_output  LeftPortType=input  RightPortType=output  PseudoPeriodic=off  Frequencies=[]  VectorFormat=1-D array  Unit=V  AffineConversion=on
  SOC_estimator : Subsystem  Commented=on
  To Workspace1 : ToWorkspace  VariableName=idc_battery_sim  SampleTime=tc
      settings: MaxDataPoints=Nc
  To Workspace2 : ToWorkspace  VariableName=udc_battery_sim  SampleTime=tc
      settings: MaxDataPoints=Nc
  Unit Delay5 : UnitDelay  SampleTime=ts_zvs  HasFrameUpgradeWarning=on
  Voltage Sensor : fl_lib/Electrical/Electrical Sensors/Voltage Sensor
  ibat/vdc : Scope  NumInputPorts=2
      settings: SampleTime=tc  ActiveDisplayYMinimum=-44.8046  ActiveDisplayYMaximum=130.4384  DataLoggingVariableName=ScopeData6
  lithium ion cell analytical ocv : Subsystem
  Uout+ : PMIOPort  Side=Right
  Uout- : PMIOPort  Port=2  Side=Right
  wires:
  PS-Simulink Converter5/1 -> Unit Delay5/1
  PS-Simulink Converter4/1 -> To Workspace1/1, ibat/vdc/1  "i batt"
  Unit Delay5/1 -> To Workspace2/1, [vdc]
  [vdc] -> ibat/vdc/2  "vdc"
  connections:
  Current Sensor/RConn1 -- PS-Simulink Converter4/LConn1
  Uout+/RConn1 -- Current Sensor/RConn2 -- Voltage Sensor/LConn1
  Voltage Sensor/RConn1 -- PS-Simulink Converter5/LConn1
  Voltage Sensor/RConn2 -- Electrical Reference1/LConn1 -- lithium ion cell analytical ocv/RConn2 -- Uout-/RConn1
  lithium ion cell analytical ocv/RConn1 -- Current Sensor/LConn1

== system three_level_sv/theee-level-inverter/three-level-inverter/stage-1 ==
  gate_commands : Inport
  Cdc1 : fl_lib/Electrical/Electrical Elements/Capacitor  c=7e-3 F  r=RCFi_dc_internal Ohm  g=0 1/Ohm  i_specify=off  i_priority=None  i=0 A  i_nominal_specify=off  i_nominal_value=1  i_nominal_unit=A  v_specify=on  v_priority=None  v=Vbattery_nom/2 V  v_nominal_specify=off  v_nominal_value=1  v_nominal_unit=V  vc_specify=off  vc_priority=High  vc=0 V  vc_nominal_specify=off  vc_nominal_value=1  vc_nominal_unit=V
  Cdc2 : fl_lib/Electrical/Electrical Elements/Capacitor  c=7e-3 F  r=RCFi_dc_internal Ohm  g=0 1/Ohm  i_specify=off  i_priority=None  i=0 A  i_nominal_specify=off  i_nominal_value=1  i_nominal_unit=A  v_specify=on  v_priority=High  v=Vbattery_nom/2 V  v_nominal_specify=off  v_nominal_value=1  v_nominal_unit=V  vc_specify=off  vc_priority=High  vc=0 V  vc_nominal_specify=off  vc_nominal_value=1  vc_nominal_unit=V
  three-level-inverter : Subsystem
  uu : PMIOPort  Side=Left
  uv : PMIOPort  Port=2  Side=Left
  Udc(+) : PMIOPort  Port=3  Side=Right
  np : PMIOPort  Port=4  Side=Right
  Udc(-) : PMIOPort  Port=5  Side=Right
  uw : PMIOPort  Port=6  Side=Left
  wires:
  gate_commands/1 -> three-level-inverter/1(gate_commands)
  connections:
  three-level-inverter/LConn1 -- uu/RConn1
  three-level-inverter/LConn2 -- uv/RConn1
  three-level-inverter/RConn1 -- Cdc1/LConn1 -- Udc(+)/RConn1
  three-level-inverter/LConn3 -- uw/RConn1
  Udc(-)/RConn1 -- three-level-inverter/RConn3 -- Cdc2/RConn1
  Cdc1/RConn1 -- np/RConn1 -- three-level-inverter/RConn2 -- Cdc2/LConn1

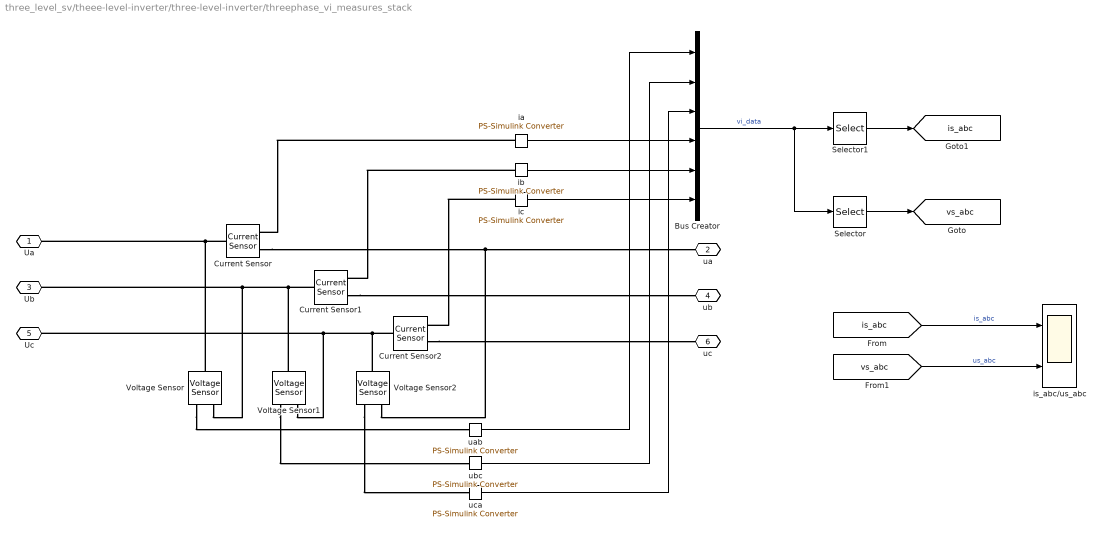
== system three_level_sv/theee-level-inverter/three-level-inverter/threephase_vi_measures_stack ==
  Bus Creator : BusCreator  Inputs=6
  Current Sensor : fl_lib/Electrical/Electrical Sensors/Current Sensor
  Current Sensor1 : fl_lib/Electrical/Electrical Sensors/Current Sensor
  Current Sensor2 : fl_lib/Electrical/Electrical Sensors/Current Sensor
  Selector : Selector  InputPortWidth=6  IndexOptions=Index vector (dialog)  Indices=[1 2 3]  OutputSizes=1
  Selector1 : Selector  InputPortWidth=6  IndexOptions=Index vector (dialog)  Indices=[4 5 6]  OutputSizes=1
  Voltage Sensor : fl_lib/Electrical/Electrical Sensors/Voltage Sensor
  Voltage Sensor1 : fl_lib/Electrical/Electrical Sensors/Voltage Sensor
  Voltage Sensor2 : fl_lib/Electrical/Electrical Sensors/Voltage Sensor
  ia : nesl_utility/PS-Simulink Converter  PhysicalDomain=network_engine_domain  SubClassName=ps_output  LeftPortType=input  RightPortType=output  PseudoPeriodic=off  Frequencies=[]  VectorFormat=1-D array  Unit=A  AffineConversion=off
  ib : nesl_utility/PS-Simulink Converter  PhysicalDomain=network_engine_domain  SubClassName=ps_output  LeftPortType=input  RightPortType=output  PseudoPeriodic=off  Frequencies=[]  VectorFormat=1-D array  Unit=A  AffineConversion=off
  ic : nesl_utility/PS-Simulink Converter  PhysicalDomain=network_engine_domain  SubClassName=ps_output  LeftPortType=input  RightPortType=output  PseudoPeriodic=off  Frequencies=[]  VectorFormat=1-D array  Unit=A  AffineConversion=off
  is_abc/us_abc : Scope  NumInputPorts=2
      settings: SampleTime=tc  ActiveDisplayYMinimum=-63.827543245438804  ActiveDisplayYMaximum=62.748196989698293
  uab : nesl_utility/PS-Simulink Converter  PhysicalDomain=network_engine_domain  SubClassName=ps_output  LeftPortType=input  RightPortType=output  PseudoPeriodic=off  Frequencies=[]  VectorFormat=1-D array  Unit=V  AffineConversion=off
  ubc : nesl_utility/PS-Simulink Converter  PhysicalDomain=network_engine_domain  SubClassName=ps_output  LeftPortType=input  RightPortType=output  PseudoPeriodic=off  Frequencies=[]  VectorFormat=1-D array  Unit=V  AffineConversion=off
  uca : nesl_utility/PS-Simulink Converter  PhysicalDomain=network_engine_domain  SubClassName=ps_output  LeftPortType=input  RightPortType=output  PseudoPeriodic=off  Frequencies=[]  VectorFormat=1-D array  Unit=V  AffineConversion=off
  Ua : PMIOPort  Side=Left
  ua : PMIOPort  Port=2  Side=Right
  Ub : PMIOPort  Port=3  Side=Left
  ub : PMIOPort  Port=4  Side=Right
  Uc : PMIOPort  Port=5  Side=Left
  uc : PMIOPort  Port=6  Side=Right
  tag scope: is_abc=global, vs_abc=global
  wires:
  Bus Creator/1 -> Selector1/1, Selector/1  "vi_data"
  Selector/1 -> [vs_abc]
  ib/1 -> Bus Creator/5
  ia/1 -> Bus Creator/4
  ic/1 -> Bus Creator/6
  Selector1/1 -> [is_abc]
  [is_abc] -> is_abc/us_abc/1  "is_abc"
  [vs_abc] -> is_abc/us_abc/2  "us_abc"
  uab/1 -> Bus Creator/1
  ubc/1 -> Bus Creator/2
  uca/1 -> Bus Creator/3
  connections:
  Current Sensor1/LConn1 -- Voltage Sensor/RConn2 -- Ub/RConn1 -- Voltage Sensor1/LConn1
  Voltage Sensor/RConn1 -- uab/LConn1
  Current Sensor/RConn2 -- Voltage Sensor2/RConn2 -- ua/RConn1
  Voltage Sensor1/RConn1 -- ubc/LConn1
  Voltage Sensor2/LConn1 -- Voltage Sensor1/RConn2 -- Uc/RConn1 -- Current Sensor2/LConn1
  Current Sensor/LConn1 -- Ua/RConn1 -- Voltage Sensor/LConn1
  Current Sensor1/RConn2 -- ub/RConn1
  Voltage Sensor2/RConn1 -- uca/LConn1
  ib/LConn1 -- Current Sensor1/RConn1
  ia/LConn1 -- Current Sensor/RConn1
  ic/LConn1 -- Current Sensor2/RConn1
  Current Sensor2/RConn2 -- uc/RConn1

== system three_level_sv/theee-level-inverter-pwm/battery_system/LithiumIonBattery ==
  Current Sensor : fl_lib/Electrical/Electrical Sensors/Current Sensor
  Electrical Reference1 : fl_lib/Electrical/Electrical Elements/Electrical Reference
  PS-Simulink Converter4 : nesl_utility/PS-Simulink Converter  PhysicalDomain=network_engine_domain  SubClassName=ps_output  LeftPortType=input  RightPortType=output  PseudoPeriodic=off  Frequencies=[]  VectorFormat=1-D array  Unit=1  AffineConversion=off
  PS-Simulink Converter5 : nesl_utility/PS-Simulink Converter  PhysicalDomain=network_engine_domain  SubClassName=ps_output  LeftPortType=input  RightPortType=output  PseudoPeriodic=off  Frequencies=[]  VectorFormat=1-D array  Unit=V  AffineConversion=on
  SOC_estimator : Subsystem  Commented=on
  To Workspace1 : ToWorkspace  VariableName=idc_battery_sim  SampleTime=tc
      settings: MaxDataPoints=Nc
  To Workspace2 : ToWorkspace  VariableName=udc_battery_sim  SampleTime=tc
      settings: MaxDataPoints=Nc
  Unit Delay5 : UnitDelay  SampleTime=ts_zvs  HasFrameUpgradeWarning=on
  Voltage Sensor : fl_lib/Electrical/Electrical Sensors/Voltage Sensor
  ibat/vdc : Scope  NumInputPorts=2
      settings: SampleTime=tc  ActiveDisplayYMinimum=-44.8046  ActiveDisplayYMaximum=130.4384  DataLoggingVariableName=ScopeData6
  lithium ion cell analytical ocv : Subsystem
  Uout+ : PMIOPort  Side=Right
  Uout- : PMIOPort  Port=2  Side=Right
  wires:
  [vdc] -> ibat/vdc/2  "vdc"
  Unit Delay5/1 -> [vdc], To Workspace2/1
  PS-Simulink Converter4/1 -> ibat/vdc/1, To Workspace1/1  "i batt"
  PS-Simulink Converter5/1 -> Unit Delay5/1
  connections:
  lithium ion cell analytical ocv/RConn1 -- Current Sensor/LConn1
  Uout-/RConn1 -- lithium ion cell analytical ocv/RConn2 -- Electrical Reference1/LConn1 -- Voltage Sensor/RConn2
  Voltage Sensor/RConn1 -- PS-Simulink Converter5/LConn1
  Voltage Sensor/LConn1 -- Current Sensor/RConn2 -- Uout+/RConn1
  Current Sensor/RConn1 -- PS-Simulink Converter4/LConn1

== system three_level_sv/theee-level-inverter-pwm/pwm_commands/PWM generator u ==
  m_index : Inport
  phase : Inport  Port=2
  Mux : Mux
  carry_n : Subsystem
  carry_p : Subsystem
  modulator_n : Subsystem
  modulator_p : Subsystem
  m : Outport
  wires:
  phase/1 -> carry_n/1(phase), carry_p/1(phase)
  carry_p/1(trp) -> modulator_p/1(tr)
  carry_n/1(trn) -> modulator_n/1(tr)
  m_index/1 -> modulator_n/2(m_index), modulator_p/2(m_index)
  modulator_p/1(m1) -> [m1]
  modulator_p/2(m3) -> [m3]
  modulator_n/1(m2) -> [m2]
  modulator_n/2(m4) -> [m4]
  [m1] -> Mux/1
  [m2] -> Mux/2
  [m3] -> Mux/3
  [m4] -> Mux/4
  Mux/1 -> m/1

== system three_level_sv/theee-level-inverter-pwm/pwm_commands/PWM generator u1 ==
  m_index : Inport
  phase : Inport  Port=2
  Mux : Mux
  carry_n : Subsystem
  carry_p : Subsystem
  modulator_n : Subsystem
  modulator_p : Subsystem
  m : Outport
  wires:
  Mux/1 -> m/1
  [m4] -> Mux/4
  [m3] -> Mux/3
  [m2] -> Mux/2
  [m1] -> Mux/1
  modulator_n/2(m4) -> [m4]
  modulator_n/1(m2) -> [m2]
  modulator_p/2(m3) -> [m3]
  modulator_p/1(m1) -> [m1]
  m_index/1 -> modulator_p/2(m_index), modulator_n/2(m_index)
  carry_n/1(trn) -> modulator_n/1(tr)
  carry_p/1(trp) -> modulator_p/1(tr)
  phase/1 -> carry_p/1(phase), carry_n/1(phase)

== system three_level_sv/theee-level-inverter-pwm/pwm_commands/PWM generator u2 ==
  m_index : Inport
  phase : Inport  Port=2
  Mux : Mux
  carry_n : Subsystem
  carry_p : Subsystem
  modulator_n : Subsystem
  modulator_p : Subsystem
  m : Outport
  wires:
  phase/1 -> carry_n/1(phase), carry_p/1(phase)
  carry_p/1(trp) -> modulator_p/1(tr)
  carry_n/1(trn) -> modulator_n/1(tr)
  m_index/1 -> modulator_n/2(m_index), modulator_p/2(m_index)
  modulator_p/1(m1) -> [m1]
  modulator_p/2(m3) -> [m3]
  modulator_n/1(m2) -> [m2]
  modulator_n/2(m4) -> [m4]
  [m1] -> Mux/1
  [m2] -> Mux/2
  [m3] -> Mux/3
  [m4] -> Mux/4
  Mux/1 -> m/1

== system three_level_sv/theee-level-inverter-pwm/three-level-inverter/stage-1 ==
  gate_commands : Inport
  Cdc1 : fl_lib/Electrical/Electrical Elements/Capacitor  c=7e-3 F  r=RCFi_dc_internal Ohm  g=0 1/Ohm  i_specify=off  i_priority=None  i=0 A  i_nominal_specify=off  i_nominal_value=1  i_nominal_unit=A  v_specify=on  v_priority=None  v=Vbattery_nom/2 V  v_nominal_specify=off  v_nominal_value=1  v_nominal_unit=V  vc_specify=off  vc_priority=High  vc=0 V  vc_nominal_specify=off  vc_nominal_value=1  vc_nominal_unit=V
  Cdc2 : fl_lib/Electrical/Electrical Elements/Capacitor  c=7e-3 F  r=RCFi_dc_internal Ohm  g=0 1/Ohm  i_specify=off  i_priority=None  i=0 A  i_nominal_specify=off  i_nominal_value=1  i_nominal_unit=A  v_specify=on  v_priority=High  v=Vbattery_nom/2 V  v_nominal_specify=off  v_nominal_value=1  v_nominal_unit=V  vc_specify=off  vc_priority=High  vc=0 V  vc_nominal_specify=off  vc_nominal_value=1  vc_nominal_unit=V
  three-level-inverter : Subsystem
  uu : PMIOPort  Side=Left
  uv : PMIOPort  Port=2  Side=Left
  Udc(+) : PMIOPort  Port=3  Side=Right
  np : PMIOPort  Port=4  Side=Right
  Udc(-) : PMIOPort  Port=5  Side=Right
  uw : PMIOPort  Port=6  Side=Left
  wires:
  gate_commands/1 -> three-level-inverter/1(gate_commands)
  connections:
  Cdc2/LConn1 -- three-level-inverter/RConn2 -- np/RConn1 -- Cdc1/RConn1
  Cdc2/RConn1 -- three-level-inverter/RConn3 -- Udc(-)/RConn1
  three-level-inverter/LConn3 -- uw/RConn1
  Udc(+)/RConn1 -- Cdc1/LConn1 -- three-level-inverter/RConn1
  three-level-inverter/LConn2 -- uv/RConn1
  three-level-inverter/LConn1 -- uu/RConn1

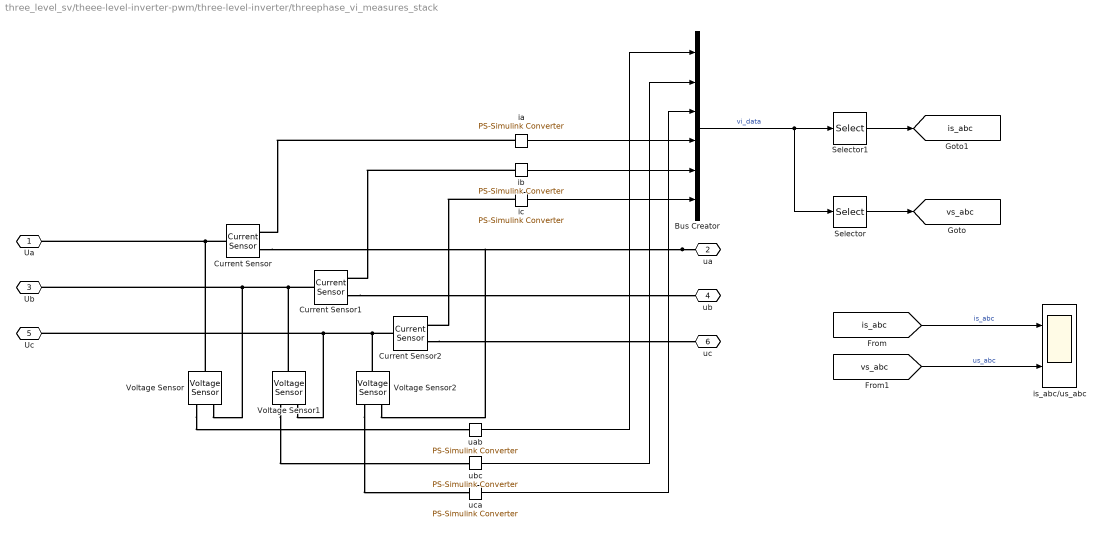
== system three_level_sv/theee-level-inverter-pwm/three-level-inverter/threephase_vi_measures_stack ==
  Bus Creator : BusCreator  Inputs=6
  Current Sensor : fl_lib/Electrical/Electrical Sensors/Current Sensor
  Current Sensor1 : fl_lib/Electrical/Electrical Sensors/Current Sensor
  Current Sensor2 : fl_lib/Electrical/Electrical Sensors/Current Sensor
  Selector : Selector  InputPortWidth=6  IndexOptions=Index vector (dialog)  Indices=[1 2 3]  OutputSizes=1
  Selector1 : Selector  InputPortWidth=6  IndexOptions=Index vector (dialog)  Indices=[4 5 6]  OutputSizes=1
  Voltage Sensor : fl_lib/Electrical/Electrical Sensors/Voltage Sensor
  Voltage Sensor1 : fl_lib/Electrical/Electrical Sensors/Voltage Sensor
  Voltage Sensor2 : fl_lib/Electrical/Electrical Sensors/Voltage Sensor
  ia : nesl_utility/PS-Simulink Converter  PhysicalDomain=network_engine_domain  SubClassName=ps_output  LeftPortType=input  RightPortType=output  PseudoPeriodic=off  Frequencies=[]  VectorFormat=1-D array  Unit=A  AffineConversion=off
  ib : nesl_utility/PS-Simulink Converter  PhysicalDomain=network_engine_domain  SubClassName=ps_output  LeftPortType=input  RightPortType=output  PseudoPeriodic=off  Frequencies=[]  VectorFormat=1-D array  Unit=A  AffineConversion=off
  ic : nesl_utility/PS-Simulink Converter  PhysicalDomain=network_engine_domain  SubClassName=ps_output  LeftPortType=input  RightPortType=output  PseudoPeriodic=off  Frequencies=[]  VectorFormat=1-D array  Unit=A  AffineConversion=off
  is_abc/us_abc : Scope  NumInputPorts=2
      settings: SampleTime=tc  ActiveDisplayYMinimum=-312.27248439804697  ActiveDisplayYMaximum=265.73282062878735
  uab : nesl_utility/PS-Simulink Converter  PhysicalDomain=network_engine_domain  SubClassName=ps_output  LeftPortType=input  RightPortType=output  PseudoPeriodic=off  Frequencies=[]  VectorFormat=1-D array  Unit=V  AffineConversion=off
  ubc : nesl_utility/PS-Simulink Converter  PhysicalDomain=network_engine_domain  SubClassName=ps_output  LeftPortType=input  RightPortType=output  PseudoPeriodic=off  Frequencies=[]  VectorFormat=1-D array  Unit=V  AffineConversion=off
  uca : nesl_utility/PS-Simulink Converter  PhysicalDomain=network_engine_domain  SubClassName=ps_output  LeftPortType=input  RightPortType=output  PseudoPeriodic=off  Frequencies=[]  VectorFormat=1-D array  Unit=V  AffineConversion=off
  Ua : PMIOPort  Side=Left
  ua : PMIOPort  Port=2  Side=Right
  Ub : PMIOPort  Port=3  Side=Left
  ub : PMIOPort  Port=4  Side=Right
  Uc : PMIOPort  Port=5  Side=Left
  uc : PMIOPort  Port=6  Side=Right
  tag scope: is_abc=global, vs_abc=global
  wires:
  uca/1 -> Bus Creator/3
  ubc/1 -> Bus Creator/2
  uab/1 -> Bus Creator/1
  [vs_abc] -> is_abc/us_abc/2  "us_abc"
  [is_abc] -> is_abc/us_abc/1  "is_abc"
  Selector1/1 -> [is_abc]
  ic/1 -> Bus Creator/6
  ia/1 -> Bus Creator/4
  ib/1 -> Bus Creator/5
  Selector/1 -> [vs_abc]
  Bus Creator/1 -> Selector/1, Selector1/1  "vi_data"
  connections:
  Current Sensor2/RConn2 -- uc/RConn1
  ic/LConn1 -- Current Sensor2/RConn1
  ia/LConn1 -- Current Sensor/RConn1
  ib/LConn1 -- Current Sensor1/RConn1
  Voltage Sensor2/RConn1 -- uca/LConn1
  Current Sensor1/RConn2 -- ub/RConn1
  Voltage Sensor/LConn1 -- Ua/RConn1 -- Current Sensor/LConn1
  Current Sensor2/LConn1 -- Uc/RConn1 -- Voltage Sensor1/RConn2 -- Voltage Sensor2/LConn1
  Voltage Sensor1/RConn1 -- ubc/LConn1
  ua/RConn1 -- Voltage Sensor2/RConn2 -- Current Sensor/RConn2
  Voltage Sensor/RConn1 -- uab/LConn1
  Voltage Sensor1/LConn1 -- Ub/RConn1 -- Voltage Sensor/RConn2 -- Current Sensor1/LConn1

== system three_level_sv/theee-level-inverter/battery_system/LithiumIonBattery/SOC_estimator ==
  Kalman_observer : Subsystem
  SOC*/SOC : Scope  Commented=on  NumInputPorts=2
      settings: SampleTime=tsample  ActiveDisplayYMinimum=-0.16149  ActiveDisplayYMaximum=0.90685
  Selector1 : Selector  InputPortWidth=3  IndexOptions=Index vector (dialog)  Indices=3  OutputSizes=1
  h_hat/h : Scope  Commented=on  NumInputPorts=2
      settings: SampleTime=tsample  ActiveDisplayYMinimum=-0.13002  ActiveDisplayYMaximum=0.15534  DataLoggingVariableName=ScopeData2
  i_out/v_out : Scope  Commented=on  NumInputPorts=2
      settings: SampleTime=tsample  ActiveDisplayYMinimum=-467.6442  ActiveDisplayYMaximum=280.8763  DataLoggingVariableName=ScopeData3
  soc/iout : Scope  Commented=on  NumInputPorts=2
      settings: SampleTime=tsample  ActiveDisplayYMinimum=0.19925  ActiveDisplayYMaximum=0.20008  DataLoggingVariableName=ScopeData4
  wires:
  Kalman_observer/2(SOC) -> SOC*/SOC/2
  Kalman_observer/1(x(k+1|k)) -> Selector1/1
  [im] -> i_out/v_out/1  "im+noise"
  [h] -> h_hat/h/2
  [SOC] -> soc/iout/1, SOC*/SOC/1
  Selector1/1 -> h_hat/h/1  "h_hat(z)"
  [vout] -> Kalman_observer/1(vout(k)), i_out/v_out/2
  [icell] -> soc/iout/2
